simulink model "thermal_closed_loop_model"  (R2023a)
settings: Solver=ode23t  StartTime=0.0  StopTime=600  RelTol=1e-3
PostLoadFcn:
  | run('thermal_model_parameters.m')
  | run('thermal_harness_parameters.m')
  | run('thermal_variants_config.m')
values from neighbouring files (symbols this model uses):
  air_cp = 1004    [cathode_subsystem_parameters.m]    (also in thermal_subsystem_parameters.m)
  air_HC_min = 10    [cathode_subsystem_parameters.m]    (also in thermal_subsystem_parameters.m)
  air_HC_nom = 100    [cathode_subsystem_parameters.m]    (also in thermal_subsystem_parameters.m)
  air_rho = 1.2    [cathode_subsystem_parameters.m]    (also in thermal_subsystem_parameters.m)
  air_vel_nom = 1    [cathode_subsystem_parameters.m]    (also in thermal_subsystem_parameters.m)
  coolant_initial_pressure = 0.111325    [cathode_subsystem_parameters.m]    (also in thermal_subsystem_parameters.m)
  coolant_initial_temperature = 293.15    [cathode_subsystem_parameters.m]    (also in thermal_subsystem_parameters.m)
  coolant_tube_D = 0.05    [cathode_subsystem_parameters.m]    (also in thermal_subsystem_parameters.m)
  Hydrowell_VTS =     [Hydrowell_values_VLV.mat]
  radiator_area_air = 0.10260000000000001    (= 0.1026)    [cathode_subsystem_parameters.m]    (also in thermal_subsystem_parameters.m)
  radiator_area_fins = 2.5436250000000005    (= 2.543625)    [cathode_subsystem_parameters.m]    (also in thermal_subsystem_parameters.m)
  radiator_area_primary = 0.44452500000000011    (= 0.444525)    [cathode_subsystem_parameters.m]    (also in thermal_subsystem_parameters.m = 2 * radiator_tube_length * radiator_width * (radiator_fin_ro)
  radiator_n_tubes = 20    [cathode_subsystem_parameters.m]    (also in thermal_subsystem_parameters.m)
  radiator_tube_height = 0.0015    [cathode_subsystem_parameters.m]    (also in thermal_subsystem_parameters.m)
  radiator_tube_length = 0.45    [cathode_subsystem_parameters.m]    (also in thermal_subsystem_parameters.m)
  radiator_width = 0.025    [cathode_subsystem_parameters.m]    (also in thermal_subsystem_parameters.m)
  tcp_time_constant = 2    [cathode_subsystem_parameters.m]    (also in thermal_subsystem_parameters.m)
undefined symbols (not defined in the file or in its folder): sigbuilder_block, stack
libraries: fl_lib x153, nesl_utility x122, SimscapeFluids_lib x16, slpidlib x5, simulink x1
(part 8 of 8)

== system thermal_closed_loop_model/Plant Model H175-Cathode-S1/Sensor LH2 in ==
  Absolute Reference (2P) : fl_lib/Two-Phase Fluid/Elements/Absolute Reference (2P)
  Mass & Energy Flow Rate Sensor (2P)1 : fl_lib/Two-Phase Fluid/Sensors/Flow Rate Sensor (2P)  mass_flow_measure=true  volumetric_flow_measure=false  energy_flow_measure=true
      settings: InternalSimscapePortConfiguration="{\"Bottom\":[{\"id\":\"PHI\",\"label\":\"φ\",\"type\":\"output\"}],\"Left\":[{\"id\":\"A\",\"label\":\"A\",\"type\":\"foundation.two_phase_fluid.two_phase_fluid\"}],\"Right\":[{\"id\":\"B\",\"label\":\"B\",\"type\":\"foundation.two_phase_fluid.two_phase_fluid\"},{\"id\":\"M\",\"label\":\"M\",\"type\":\"output\"}],\"Top\":[]}"
  PS-Simulink Converter : nesl_utility/PS-Simulink Converter  PhysicalDomain=network_engine_domain  SubClassName=ps_output  LeftPortType=input  RightPortType=output  PseudoPeriodic=off  Frequencies=[]  VectorFormat=inherit  Unit=kW  AffineConversion=off
  PS-Simulink Converter1 : nesl_utility/PS-Simulink Converter  PhysicalDomain=network_engine_domain  SubClassName=ps_output  LeftPortType=input  RightPortType=output  PseudoPeriodic=off  Frequencies=[]  VectorFormat=1-D array  Unit=inherit  AffineConversion=off
  PS-Simulink Converter2 : nesl_utility/PS-Simulink Converter  PhysicalDomain=network_engine_domain  SubClassName=ps_output  LeftPortType=input  RightPortType=output  PseudoPeriodic=off  Frequencies=[]  VectorFormat=1-D array  Unit=inherit  AffineConversion=off
  PS-Simulink Converter3 : nesl_utility/PS-Simulink Converter  PhysicalDomain=network_engine_domain  SubClassName=ps_output  LeftPortType=input  RightPortType=output  PseudoPeriodic=off  Frequencies=[]  VectorFormat=1-D array  Unit=inherit  AffineConversion=off
  Pressure & Internal Energy Sensor (2P) : fl_lib/Two-Phase Fluid/Sensors/Pressure, Temperature & Internal Energy Sensor (2P)  reference=foundation.enum.MeasurementReference.difference  pressure=true  pressure_spec=foundation.enum.PressureMeasementSpec.Absolute  temperature=false  internal_energy=true
      settings: InternalSimscapePortConfiguration="{\"Bottom\":[{\"id\":\"U\",\"label\":\"U\",\"type\":\"output\"}],\"Left\":[{\"id\":\"A\",\"label\":\"A\",\"type\":\"foundation.two_phase_fluid.two_phase_fluid\"}],\"Right\":[{\"id\":\"B\",\"label\":\"B\",\"type\":\"foundation.two_phase_fluid.two_phase_fluid\"},{\"id\":\"P\",\"label\":\"P\",\"type\":\"output\"}],\"Top\":[]}"
  Thermodynamic Properties Sensor (2P) : fl_lib/Two-Phase Fluid/Sensors/Thermodynamic Properties Sensor (2P)  temperature=true  enthalpy=true  density=false  specific_volume=true  entropy=true
      settings: InternalSimscapePortConfiguration="{\"Bottom\":[{\"id\":\"V\",\"label\":\"v\",\"type\":\"output\"},{\"id\":\"S\",\"label\":\"s\",\"type\":\"output\"}],\"Left\":[{\"id\":\"A\",\"label\":\"A\",\"type\":\"foundation.two_phase_fluid.two_phase_fluid\"}],\"Right\":[{\"id\":\"T\",\"label\":\"T\",\"type\":\"output\"},{\"id\":\"H\",\"label\":\"h\",\"type\":\"output\"}],\"Top\":[]}"
  A : PMIOPort  Side=Left
  B : PMIOPort  Port=2  Side=Right
  tag scope: S5_Energy=global, S5_Temp=global, S5_aPres=global, S5_mFLow=global
  wires:
  PS-Simulink Converter3/1 -> [S5_mFLow]
  PS-Simulink Converter2/1 -> [S5_aPres]
  PS-Simulink Converter1/1 -> [S5_Temp]
  PS-Simulink Converter/1 -> [S5_Energy]
  connections:
  Pressure & Internal Energy Sensor (2P)/RConn1 -- Absolute Reference (2P)/LConn1
  Mass & Energy Flow Rate Sensor (2P)1/RConn2 -- PS-Simulink Converter3/LConn1
  PS-Simulink Converter2/LConn1 -- Pressure & Internal Energy Sensor (2P)/RConn2
  Thermodynamic Properties Sensor (2P)/RConn1 -- PS-Simulink Converter1/LConn1
  Mass & Energy Flow Rate Sensor (2P)1/RConn3 -- PS-Simulink Converter/LConn1
  Mass & Energy Flow Rate Sensor (2P)1/LConn1 -- Pressure & Internal Energy Sensor (2P)/LConn1 -- Thermodynamic Properties Sensor (2P)/LConn1 -- A/RConn1
  Mass & Energy Flow Rate Sensor (2P)1/RConn1 -- B/RConn1

== system thermal_closed_loop_model/Plant Model H175-Cathode-S1/Sensor LH2 out ==
  Absolute Reference (2P) : fl_lib/Two-Phase Fluid/Elements/Absolute Reference (2P)
  Mass & Energy Flow Rate Sensor (2P)1 : fl_lib/Two-Phase Fluid/Sensors/Flow Rate Sensor (2P)  mass_flow_measure=true  volumetric_flow_measure=false  energy_flow_measure=true
      settings: InternalSimscapePortConfiguration="{\"Bottom\":[{\"id\":\"PHI\",\"label\":\"φ\",\"type\":\"output\"}],\"Left\":[{\"id\":\"A\",\"label\":\"A\",\"type\":\"foundation.two_phase_fluid.two_phase_fluid\"}],\"Right\":[{\"id\":\"B\",\"label\":\"B\",\"type\":\"foundation.two_phase_fluid.two_phase_fluid\"},{\"id\":\"M\",\"label\":\"M\",\"type\":\"output\"}],\"Top\":[]}"
  PS-Simulink Converter : nesl_utility/PS-Simulink Converter  PhysicalDomain=network_engine_domain  SubClassName=ps_output  LeftPortType=input  RightPortType=output  PseudoPeriodic=off  Frequencies=[]  VectorFormat=1-D array  Unit=kW  AffineConversion=off
  PS-Simulink Converter1 : nesl_utility/PS-Simulink Converter  PhysicalDomain=network_engine_domain  SubClassName=ps_output  LeftPortType=input  RightPortType=output  PseudoPeriodic=off  Frequencies=[]  VectorFormat=1-D array  Unit=degC  AffineConversion=off
  PS-Simulink Converter2 : nesl_utility/PS-Simulink Converter  PhysicalDomain=network_engine_domain  SubClassName=ps_output  LeftPortType=input  RightPortType=output  PseudoPeriodic=off  Frequencies=[]  VectorFormat=1-D array  Unit=1  AffineConversion=off
  PS-Simulink Converter3 : nesl_utility/PS-Simulink Converter  PhysicalDomain=network_engine_domain  SubClassName=ps_output  LeftPortType=input  RightPortType=output  PseudoPeriodic=off  Frequencies=[]  VectorFormat=1-D array  Unit=inherit  AffineConversion=off
  Pressure & Internal Energy Sensor (2P) : fl_lib/Two-Phase Fluid/Sensors/Pressure, Temperature & Internal Energy Sensor (2P)  reference=foundation.enum.MeasurementReference.difference  pressure=true  pressure_spec=foundation.enum.PressureMeasementSpec.Absolute  temperature=false  internal_energy=true
      settings: InternalSimscapePortConfiguration="{\"Bottom\":[{\"id\":\"U\",\"label\":\"U\",\"type\":\"output\"}],\"Left\":[{\"id\":\"A\",\"label\":\"A\",\"type\":\"foundation.two_phase_fluid.two_phase_fluid\"}],\"Right\":[{\"id\":\"B\",\"label\":\"B\",\"type\":\"foundation.two_phase_fluid.two_phase_fluid\"},{\"id\":\"P\",\"label\":\"P\",\"type\":\"output\"}],\"Top\":[]}"
  Thermodynamic Properties Sensor (2P) : fl_lib/Two-Phase Fluid/Sensors/Thermodynamic Properties Sensor (2P)  temperature=true  enthalpy=true  density=false  specific_volume=true  entropy=true
      settings: InternalSimscapePortConfiguration="{\"Bottom\":[{\"id\":\"V\",\"label\":\"v\",\"type\":\"output\"},{\"id\":\"S\",\"label\":\"s\",\"type\":\"output\"}],\"Left\":[{\"id\":\"A\",\"label\":\"A\",\"type\":\"foundation.two_phase_fluid.two_phase_fluid\"}],\"Right\":[{\"id\":\"T\",\"label\":\"T\",\"type\":\"output\"},{\"id\":\"H\",\"label\":\"h\",\"type\":\"output\"}],\"Top\":[]}"
  A : PMIOPort  Side=Left
  B : PMIOPort  Port=2  Side=Right
  tag scope: S6_Energy=global, S6_Temp=global, S6_aPres=global, S6_mFlow=global
  wires:
  PS-Simulink Converter3/1 -> [S6_aPres]
  PS-Simulink Converter2/1 -> [S6_mFlow]
  PS-Simulink Converter/1 -> [S6_Energy]
  PS-Simulink Converter1/1 -> [S6_Temp]
  connections:
  Pressure & Internal Energy Sensor (2P)/RConn1 -- Absolute Reference (2P)/LConn1
  Mass & Energy Flow Rate Sensor (2P)1/LConn1 -- Pressure & Internal Energy Sensor (2P)/LConn1 -- Thermodynamic Properties Sensor (2P)/LConn1 -- A/RConn1
  Pressure & Internal Energy Sensor (2P)/RConn2 -- PS-Simulink Converter3/LConn1
  Mass & Energy Flow Rate Sensor (2P)1/RConn2 -- PS-Simulink Converter2/LConn1
  Thermodynamic Properties Sensor (2P)/RConn1 -- PS-Simulink Converter1/LConn1
  Mass & Energy Flow Rate Sensor (2P)1/RConn1 -- B/RConn1
  Mass & Energy Flow Rate Sensor (2P)1/RConn3 -- PS-Simulink Converter/LConn1

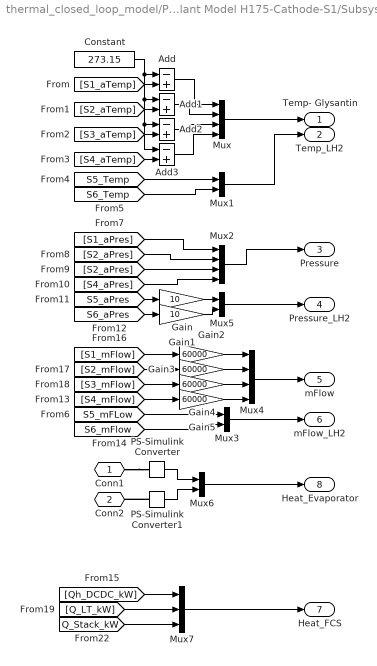
== system thermal_closed_loop_model/Plant Model H175-Cathode-S1/Subsystem4 ==
  Add{,1..3} (4 alike) : Sum  Inputs=-+
  Constant : Constant  Value=273.15
  Gain : Gain  Gain=10
  Gain1 : Gain  Gain=10
  Gain{2..5} (4 alike) : Gain  Gain=60000
  Mux : Mux
  Mux{1,3,5..6} (4 alike) : Mux  Inputs=2
  Mux2 : Mux
  Mux4 : Mux
  Mux7 : Mux  Inputs=3
  PS-Simulink Converter : nesl_utility/PS-Simulink Converter  PhysicalDomain=network_engine_domain  SubClassName=ps_output  LeftPortType=input  RightPortType=output  PseudoPeriodic=off  Frequencies=[]  VectorFormat=inherit  Unit=inherit  AffineConversion=off
  PS-Simulink Converter1 : nesl_utility/PS-Simulink Converter  PhysicalDomain=network_engine_domain  SubClassName=ps_output  LeftPortType=input  RightPortType=output  PseudoPeriodic=off  Frequencies=[]  VectorFormat=inherit  Unit=inherit  AffineConversion=off
  Conn1 : PMIOPort  Side=Left
  Conn2 : PMIOPort  Port=2  Side=Left
  Temp- Glysantin : Outport
  Temp_LH2 : Outport  Port=2
  Pressure : Outport  Port=3
  Pressure_LH2 : Outport  Port=4
  mFlow : Outport  Port=5
  mFlow_LH2 : Outport  Port=6
  Heat_FCS : Outport  Port=7
  Heat_Evaporator : Outport  Port=8
  wires:
  Mux7/1 -> Heat_FCS/1
  [Q_Stack_kW] -> Mux7/3
  [Q_LT_kW] -> Mux7/2
  [Qh_DCDC_kW] -> Mux7/1
  Mux6/1 -> Heat_Evaporator/1
  PS-Simulink Converter1/1 -> Mux6/2
  PS-Simulink Converter/1 -> Mux6/1
  Gain5/1 -> Mux4/4
  Gain4/1 -> Mux4/3
  Gain3/1 -> Mux4/2
  Gain2/1 -> Mux4/1
  Gain1/1 -> Mux5/2
  Gain/1 -> Mux5/1
  [S5_aPres] -> Gain/1
  Mux5/1 -> Pressure_LH2/1
  [S6_aPres] -> Gain1/1
  Mux3/1 -> mFlow_LH2/1
  [S5_mFLow] -> Mux3/1
  Add/1 -> Mux/1
  Add1/1 -> Mux/2
  Add2/1 -> Mux/3
  Add3/1 -> Mux/4
  [S5_Temp] -> Mux1/1
  [S6_Temp] -> Mux1/2
  [S4_aTemp] -> Add3/2
  [S3_aTemp] -> Add2/2
  [S2_aTemp] -> Add1/2
  Constant/1 -> Add/1, Add1/1, Add2/1, Add3/1
  [S1_aTemp] -> Add/2
  Mux2/1 -> Pressure/1
  Mux1/1 -> Temp_LH2/1
  Mux/1 -> Temp- Glysantin/1
  Mux4/1 -> mFlow/1
  [S6_mFlow] -> Mux3/2
  [S1_aPres] -> Mux2/1
  [S4_mFlow] -> Gain5/1
  [S2_aPres] -> Mux2/2
  [S3_mFlow] -> Gain4/1
  [S2_aPres] -> Mux2/3
  [S1_mFlow] -> Gain2/1
  [S2_mFlow] -> Gain3/1
  [S4_aPres] -> Mux2/4
  connections:
  PS-Simulink Converter1/LConn1 -- Conn2/RConn1
  Conn1/RConn1 -- PS-Simulink Converter/LConn1

== system thermal_closed_loop_model/Plant_Sensors1/EAC_Theo_Power ==
  <mFlow_S1> : Inport
  <aPres_S1> : Inport  Port=2
  <aPres_S2> : Inport  Port=3
  <aTemp_S1> : Inport  Port=4
  Cp : Constant  Value=1004
  Divide : Product  Inputs=*/
  MATLAB Function : MATLAB Function  TreatAsAtomicUnit=on
  Product : Product  Inputs=4
  y-exp : Constant  Value=(1.33-1)/1.33
  Out1 : Outport
  wires:
  Cp/1 -> Product/1
  <aTemp_S1>/1 -> Product/2
  <aPres_S1>/1 -> Divide/2
  Product/1 -> Out1/1
  <aPres_S2>/1 -> Divide/1
  MATLAB Function/1(y) -> Product/4
  y-exp/1 -> MATLAB Function/2(data)
  Divide/1 -> MATLAB Function/1(u)
  <mFlow_S1>/1 -> Product/3

== system thermal_closed_loop_model/Plant_Sensors1/EAT_Theo_Power ==
  <mFlow_S1> : Inport
  <aPres_S6> : Inport  Port=2
  <aTemp_S6> : Inport  Port=3
  <aPres_S7> : Inport  Port=4
  Cp : Constant  Value=1150
  Divide : Product  Inputs=*/
  Gain : Gain  Gain=-1
  MATLAB Function : MATLAB Function  TreatAsAtomicUnit=on
  Product : Product  Inputs=4
  y-exp : Constant  Value=(1.33-1)/1.33
  Out1 : Outport
  wires:
  y-exp/1 -> MATLAB Function/2(data)
  <aPres_S7>/1 -> Divide/1
  Cp/1 -> Product/4
  Divide/1 -> MATLAB Function/1(u)
  Product/1 -> Gain/1
  <mFlow_S1>/1 -> Product/2
  MATLAB Function/1(y) -> Product/1
  <aTemp_S6>/1 -> Product/3
  <aPres_S6>/1 -> Divide/2
  Gain/1 -> Out1/1

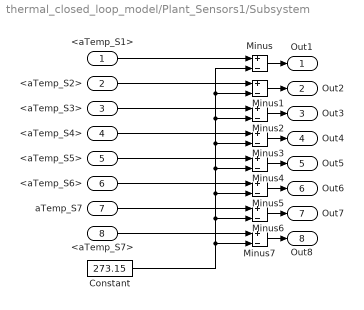
== system thermal_closed_loop_model/Plant_Sensors1/Subsystem ==
  <aTemp_S1> : Inport
  <aTemp_S2> : Inport  Port=2
  <aTemp_S3> : Inport  Port=3
  <aTemp_S4> : Inport  Port=4
  <aTemp_S5> : Inport  Port=5
  <aTemp_S6> : Inport  Port=6
  aTemp_S7 : Inport  Port=7
  <aTemp_S7> : Inport  Port=8
  Constant : Constant  Value=273.15
  Minus{,1..7} (8 alike) : Sum  Inputs=+-
  Out1 : Outport
  Out2 : Outport  Port=2
  Out3 : Outport  Port=3
  Out4 : Outport  Port=4
  Out5 : Outport  Port=5
  Out6 : Outport  Port=6
  Out7 : Outport  Port=7
  Out8 : Outport  Port=8
  wires:
  Minus4/1 -> Out5/1
  Constant/1 -> Minus7/2, Minus3/2, Minus2/2, Minus1/2, Minus/2, Minus4/2, Minus5/2, Minus6/2
  Minus2/1 -> Out3/1
  <aTemp_S7>/1 -> Minus7/1
  <aTemp_S4>/1 -> Minus3/1
  <aTemp_S1>/1 -> Minus/1
  Minus5/1 -> Out6/1
  Minus6/1 -> Out7/1
  <aTemp_S3>/1 -> Minus2/1
  Minus/1 -> Out1/1
  <aTemp_S5>/1 -> Minus4/1
  Minus3/1 -> Out4/1
  Minus1/1 -> Out2/1
  <aTemp_S6>/1 -> Minus5/1
  <aTemp_S2>/1 -> Minus1/1
  Minus7/1 -> Out8/1
  aTemp_S7/1 -> Minus6/1

== system thermal_closed_loop_model/Basic Peripherals/Variant Subsystem/Controlled_Power_HeatExchanger ==
  note: Lafer-style heat exchanger
  Environment_Temperature_K : Inport
  Heat_Flux_W : Inport  Port=2
  Controlled Temperature Source : fl_lib/Thermal/Thermal Sources/Controlled Temperature Source
  Controlled Heat Flow Rate Source : fl_lib/Thermal/Thermal Sources/Controlled Heat Flow Rate Source
  Gain : Gain  Gain=-1
  Heat Exchanger Interface (TL) : SimscapeFluids_lib/Fluid Network Interfaces/Heat Exchangers/Fundamental Components/Heat Exchanger Interface (TL)  min_flow_area=radiator_n_tubes*(radiator_width*radiator_tube_height) m^2  Dh_press=4*(radiator_width*radiator_tube_height)/(2 * (radiator_width+radiator_tube_height)) m  liquid_volume=radiator_n_tubes*(radiator_width*radiator_tube_height)*radiator_tube_length m^3  Re_lam=2000  Re_tur=4000.  pressure_loss_spec=fluids.interfaces.enum.pressure_loss_spec.tube_correlation  pressure_loss_coeff=0.1  length_press=radiator_tube_length m  length_add=0.1 m  roughness=15e-6 m  Re_friction_TLU=[400, 1000, 1500, 3000, 4000, 6000, 10000, 20000, 40000, 60000, 100000, 100000000]  friction_factor_TLU=[.264, .112, .071, .0417, .0387, .0268, .025, .0232, .0226, .022, .0214, .0214]  shape_factor=64  Re_Euler_TLU=[50, 500, 1000, 2000]  Euler_TLU=[4.4505, .6864, .4791, .3755]  heat_transfer_spec=fluids.interfaces.enum.heat_transfer_spec.tube_correlation  heat_coeff=100 W/(K*m^2)  heat_transfer_area=radiator_n_tubes*2*(radiator_tube_length*radiator_width+radiator_tube_length*radiator_tube_height) m^2  Nu_lam=3.66  Re_Colburn_TLU=[100, 150, 1000]  Colburn_factor_TLU=[.019, .013, .002]  Re_Nu_TLU=[100, 150, 1000]  Pr_Nu_TLU=[1, 10]  Nu_TLU=[3.72, 4.21; 3.75, 4.44; 4.21, 7.15]  length_heat=radiator_tube_length m  dynamic_compressibility=simscape.enum.onoff.on  T0=coolant_initial_temperature K  p0=coolant_initial_pressure MPa
      settings: InternalSimscapePortConfiguration="{\"Bottom\":[],\"Left\":[{\"id\":\"A\",\"label\":\"A\",\"type\":\"foundation.thermal_liquid.thermal_liquid\"},{\"id\":\"B\",\"label\":\"B\",\"type\":\"foundation.thermal_liquid.thermal_liquid\"}],\"Right\":[{\"id\":\"H\",\"label\":\"H\",\"type\":\"foundation.thermal.thermal\"},{\"id\":\"C\",\"label\":\"C\",\"type\":\"output\"},{\"id\":\"HC\",\"label\":\"HC\",\"type\":\"output\"}],\"Top\":[]}"
  PS Terminator : fl_lib/Physical Signals/Sinks/PS Terminator
  PS Terminator1 : fl_lib/Physical Signals/Sinks/PS Terminator
  Saturation : Saturate  UpperLimit=0  LowerLimit=-200e3
  Simulink-PS Converter3 : nesl_utility/Simulink-PS Converter  PhysicalDomain=network_engine_domain  SubClassName=ps_input  LeftPortType=input  RightPortType=output  PseudoPeriodic=off  Frequencies=[]  NoiseDistribution=none  NoiseParameters=[]  Unit=1  AffineConversion=off  FilteringAndDerivatives=provide  SimscapeFilterOrder=1  InputFilterTimeConstant=0.001  UdotUserProvided=0
  Simulink-PS Converter5 : nesl_utility/Simulink-PS Converter  PhysicalDomain=network_engine_domain  SubClassName=ps_input  LeftPortType=input  RightPortType=output  PseudoPeriodic=off  Frequencies=[]  NoiseDistribution=none  NoiseParameters=[]  Unit=1  AffineConversion=off  FilteringAndDerivatives=provide  SimscapeFilterOrder=1  InputFilterTimeConstant=0.001  UdotUserProvided=0
  Thermal Reference : fl_lib/Thermal/Thermal Elements/Thermal Reference
  Coolant_to_HeatExchanger : PMIOPort  Side=Right
  Coolant_from_HeatExchanger : PMIOPort  Port=2  Side=Right
  wires:
  Environment_Temperature_K/1 -> Simulink-PS Converter5/1
  Heat_Flux_W/1 -> Gain/1
  Gain/1 -> Saturation/1
  Saturation/1 -> Simulink-PS Converter3/1
  connections:
  Coolant_to_HeatExchanger/RConn1 -- Heat Exchanger Interface (TL)/LConn1
  PS Terminator/LConn1 -- Heat Exchanger Interface (TL)/RConn2
  Controlled Heat Flow Rate Source/RConn2 -- Controlled Temperature Source/LConn1
  Controlled Temperature Source/RConn2 -- Thermal Reference/LConn1
  Controlled Heat Flow Rate Source/LConn1 -- Heat Exchanger Interface (TL)/RConn1
  Simulink-PS Converter3/RConn1 -- Controlled Heat Flow Rate Source/RConn1
  PS Terminator1/LConn1 -- Heat Exchanger Interface (TL)/RConn3
  Simulink-PS Converter5/RConn1 -- Controlled Temperature Source/RConn1
  Coolant_from_HeatExchanger/RConn1 -- Heat Exchanger Interface (TL)/LConn2

== system thermal_closed_loop_model/Basic Peripherals/Variant Subsystem/Controlled_Temperature_HeatExchanger ==
  note: Lafer-style heat exchanger
  T_TCVi_ref_degC : Inport
  Controlled Temperature Source : fl_lib/Thermal/Thermal Sources/Controlled Temperature Source
  Controlled Heat Flow Rate Source : fl_lib/Thermal/Thermal Sources/Controlled Heat Flow Rate Source
  Gain : Gain  Gain=-20e3
  Heat Exchanger Interface (TL) : SimscapeFluids_lib/Fluid Network Interfaces/Heat Exchangers/Fundamental Components/Heat Exchanger Interface (TL)  min_flow_area=radiator_n_tubes*(radiator_width*radiator_tube_height) m^2  Dh_press=4*(radiator_width*radiator_tube_height)/(2 * (radiator_width+radiator_tube_height)) m  liquid_volume=radiator_n_tubes*(radiator_width*radiator_tube_height)*radiator_tube_length m^3  Re_lam=2000  Re_tur=4000.  pressure_loss_spec=fluids.interfaces.enum.pressure_loss_spec.tube_correlation  pressure_loss_coeff=0.1  length_press=radiator_tube_length m  length_add=0.1 m  roughness=15e-6 m  Re_friction_TLU=[400, 1000, 1500, 3000, 4000, 6000, 10000, 20000, 40000, 60000, 100000, 100000000]  friction_factor_TLU=[.264, .112, .071, .0417, .0387, .0268, .025, .0232, .0226, .022, .0214, .0214]  shape_factor=64  Re_Euler_TLU=[50, 500, 1000, 2000]  Euler_TLU=[4.4505, .6864, .4791, .3755]  heat_transfer_spec=fluids.interfaces.enum.heat_transfer_spec.tube_correlation  heat_coeff=100 W/(K*m^2)  heat_transfer_area=radiator_n_tubes*2*(radiator_tube_length*radiator_width+radiator_tube_length*radiator_tube_height) m^2  Nu_lam=3.66  Re_Colburn_TLU=[100, 150, 1000]  Colburn_factor_TLU=[.019, .013, .002]  Re_Nu_TLU=[100, 150, 1000]  Pr_Nu_TLU=[1, 10]  Nu_TLU=[3.72, 4.21; 3.75, 4.44; 4.21, 7.15]  length_heat=radiator_tube_length m  dynamic_compressibility=simscape.enum.onoff.on  T0=coolant_initial_temperature K  p0=coolant_initial_pressure MPa
      settings: InternalSimscapePortConfiguration="{\"Bottom\":[],\"Left\":[{\"id\":\"A\",\"label\":\"A\",\"type\":\"foundation.thermal_liquid.thermal_liquid\"},{\"id\":\"B\",\"label\":\"B\",\"type\":\"foundation.thermal_liquid.thermal_liquid\"}],\"Right\":[{\"id\":\"H\",\"label\":\"H\",\"type\":\"foundation.thermal.thermal\"},{\"id\":\"C\",\"label\":\"C\",\"type\":\"output\"},{\"id\":\"HC\",\"label\":\"HC\",\"type\":\"output\"}],\"Top\":[]}"
  PS Terminator : fl_lib/Physical Signals/Sinks/PS Terminator
  PS Terminator1 : fl_lib/Physical Signals/Sinks/PS Terminator
  PS-Simulink Converter : nesl_utility/PS-Simulink Converter  PhysicalDomain=network_engine_domain  SubClassName=ps_output  LeftPortType=input  RightPortType=output  PseudoPeriodic=off  Frequencies=[]  VectorFormat=inherit  Unit=inherit  AffineConversion=off
  Pressure & Temperature Sensor (TL)1 : fl_lib/Thermal Liquid/Sensors/Pressure & Temperature Sensor (TL)  reference=foundation.enum.MeasurementReference.absolute  pressure=false  pressure_spec=foundation.enum.PressureMeasementSpec.Absolute  temperature=true
      settings: InternalSimscapePortConfiguration="{\"Bottom\":[{\"id\":\"T\",\"label\":\"T\",\"type\":\"output\"}],\"Left\":[{\"id\":\"A\",\"label\":\"A\",\"type\":\"foundation.thermal_liquid.thermal_liquid\"}],\"Right\":[],\"Top\":[]}"
  Saturation : Saturate  UpperLimit=0  LowerLimit=-200e3
  Simulink-PS Converter3 : nesl_utility/Simulink-PS Converter  PhysicalDomain=network_engine_domain  SubClassName=ps_input  LeftPortType=input  RightPortType=output  PseudoPeriodic=off  Frequencies=[]  NoiseDistribution=none  NoiseParameters=[]  Unit=1  AffineConversion=off  FilteringAndDerivatives=provide  SimscapeFilterOrder=1  InputFilterTimeConstant=0.001  UdotUserProvided=0
  Simulink-PS Converter5 : nesl_utility/Simulink-PS Converter  PhysicalDomain=network_engine_domain  SubClassName=ps_input  LeftPortType=input  RightPortType=output  PseudoPeriodic=off  Frequencies=[]  NoiseDistribution=none  NoiseParameters=[]  Unit=1  AffineConversion=off  FilteringAndDerivatives=provide  SimscapeFilterOrder=1  InputFilterTimeConstant=0.001  UdotUserProvided=0
  Sum : Sum  Inputs=|+-
  Thermal Reference : fl_lib/Thermal/Thermal Elements/Thermal Reference
  Unit Delay17 : UnitDelay  SampleTime=-1  HasFrameUpgradeWarning=on
  °C to Kelvin : Subsystem
  Coolant_to_HeatExchanger : PMIOPort  Side=Right
  Coolant_from_HeatExchanger : PMIOPort  Port=2  Side=Right
  tag scope: T_TCVi_ref_degC=global
  wires:
  PS-Simulink Converter/1 -> Sum/1
  Gain/1 -> Unit Delay17/1
  Unit Delay17/1 -> Saturation/1
  T_TCVi_ref_degC/1 -> [T_TCVi_ref_degC], °C to Kelvin/1(Temp. (°C))
  Sum/1 -> Gain/1
  Saturation/1 -> Simulink-PS Converter3/1
  °C to Kelvin/1(Temp. (K)) -> Simulink-PS Converter5/1, Sum/2  "Stack Inlet Temperature: TSens_CLSti 6812 (°C)"
  connections:
  Coolant_from_HeatExchanger/RConn1 -- Pressure & Temperature Sensor (TL)1/LConn1 -- Heat Exchanger Interface (TL)/LConn2
  Simulink-PS Converter5/RConn1 -- Controlled Temperature Source/RConn1
  PS Terminator1/LConn1 -- Heat Exchanger Interface (TL)/RConn3
  Simulink-PS Converter3/RConn1 -- Controlled Heat Flow Rate Source/RConn1
  Controlled Heat Flow Rate Source/LConn1 -- Heat Exchanger Interface (TL)/RConn1
  Controlled Temperature Source/RConn2 -- Thermal Reference/LConn1
  PS-Simulink Converter/LConn1 -- Pressure & Temperature Sensor (TL)1/RConn1
  Controlled Heat Flow Rate Source/RConn2 -- Controlled Temperature Source/LConn1
  PS Terminator/LConn1 -- Heat Exchanger Interface (TL)/RConn2
  Heat Exchanger Interface (TL)/LConn1 -- Coolant_to_HeatExchanger/RConn1

== system thermal_closed_loop_model/Basic Peripherals/Variant Subsystem/Phyiscal_Radiator_Model ==
  note: Basic Radiator Model
  Convective_Airspeed_mps : Inport
  Environment_Temperature_K : Inport  Port=2
  Aircraft Duct : Subsystem
  Radiator : SimscapeFluids_lib/Fluid Network Interfaces/Heat Exchangers/Heat Exchanger (TL)  hex_type=3  shell_num=1  cross_type=4  NTU_TLU=[0.5, 1.0, 2.0, 3.0, 4.0, 5.0]  CR_TLU=[0.0, 0.25, 0.5, 0.75, 1.0]  eff_TLU=[0.3, 0.3, 0.3, 0.3, 0.3; 0.6, 0.55, 0.5, 0.47, 0.43; 0.85, 0.76, 0.68, 0.61, 0.55; 0.94, 0.83, 0.72, 0.65, 0.58; 0.98, 0.86, 0.75, 0.66, 0.58; 0.99, 0.86, 0.75, 0.66, 0.58]  R_wall=0.014/(381*radiator_n_tubes*radiator_width*radiator_tube_length) K/W  min_flow_area_1=radiator_n_tubes*(radiator_width*radiator_tube_height) m^2  Dh_press_1=4*(radiator_width*radiator_tube_height)/(2 * (radiator_width+radiator_tube_height)) m  liquid_volume_1=radiator_n_tubes*(radiator_width*radiator_tube_height)*radiator_tube_length m^3  Re_lam_1=2000  Re_tur_1=4000  pressure_loss_spec_1=fluids.interfaces.enum.pressure_loss_spec.tube_correlation  pressure_loss_coeff_1=15  length_press_1=radiator_tube_length m  length_add_1=0.1 m  roughness_1=15e-6 m  Re_friction_TLU_1=[400.0, 1000.0, 1500.0, 3000.0, 4000.0, 6000.0, 10000.0, 20000.0, 40000.0, 60000.0, 100000.0, 100000000.0]  friction_factor_TLU_1=[0.264, 0.112, 0.071, 0.0417, 0.0387, 0.0268, 0.025, 0.0232, 0.0226, 0.022, 0.0214, 0.0214]  shape_factor_1=64  Re_Euler_TLU_1=[50.0, 500.0, 1000.0, 2000.0]  Euler_TLU_1=[4.4505, 0.6864, 0.4791, 0.3755]  heat_transfer_spec_1=2  heat_transfer_area_1=radiator_n_tubes*2*(radiator_tube_length*radiator_width+radiator_tube_length*radiator_tube_height) m^2  heat_coeff_1=2000 W/(m^2 * K)  length_heat_1=radiator_tube_length cm  Nu_lam_1=3.66  Re_Colburn_TLU_1=[100.0, 150.0, 1000.0]  Colburn_factor_TLU_1=[0.019, 0.013, 0.002]  Re_Nu_TLU_1=[100.0, 150.0, 1000.0]  Pr_Nu_TLU_1=[1.0, 10.0]  Nu_TLU_1=[3.72, 4.21; 3.75, 4.44; 4.21, 7.15]  fouling_factor_1=0 m^2*K/W  min_heat_coeff_1=5 W/(m^2 * K)  heat_transfer_area_2=radiator_area_primary+radiator_area_fins m^2  fouling_factor_2=0 m^2*K/W  min_heat_coeff_2=0.01 W/(m^2 * K)  dynamic_compressibility_1=1  T0_1=coolant_initial_temperature K  p0_1=coolant_initial_pressure MPa  mdot1_TLU=[.1, .2] kg/s  mdot2_TLU=[.2, .3] kg/s  SD_TLU=[35, 35; 50, 50] kW/K  Q_check=1  mdot_dp_TLU_1=[.1, .2] kg/s  p_diff_TLU_1=[.003, .005] MPa  T_ref_in_1=293.15 K  p_ref_in_1=0.101325 MPa  mdot_threshold_1=1e-3 kg/s  area_1=0.01 m^2
      settings: InternalSimscapePortConfiguration="{\"Bottom\":[],\"Left\":[{\"id\":\"A1\",\"label\":\"A1\",\"type\":\"foundation.thermal_liquid.thermal_liquid\"},{\"id\":\"B1\",\"label\":\"B1\",\"type\":\"foundation.thermal_liquid.thermal_liquid\"}],\"Right\":[{\"id\":\"H2\",\"label\":\"H2\",\"type\":\"foundation.thermal.thermal\"},{\"id\":\"C2\",\"label\":\"C2\",\"type\":\"input\"},{\"id\":\"HC2\",\"label\":\"HC2\",\"type\":\"input\"}],\"Top\":[]}"
  Coolant_to_HeatExchanger : PMIOPort  Side=Right
  Coolant_from_HeatExchanger : PMIOPort  Port=2  Side=Right
  wires:
  Environment_Temperature_K/1 -> Aircraft Duct/2(T_air)
  Convective_Airspeed_mps/1 -> Aircraft Duct/1(V_air)
  connections:
  Radiator/RConn1 -- Aircraft Duct/RConn1
  Radiator/RConn2 -- Aircraft Duct/RConn2
  Radiator/LConn1 -- Coolant_to_HeatExchanger/RConn1
  Radiator/RConn3 -- Aircraft Duct/RConn3
  Coolant_from_HeatExchanger/RConn1 -- Radiator/LConn2

== system thermal_closed_loop_model/Fast Controller/CHU-Dry side control/Cathode Humidifier ==
  Controlled Moisture Source (MA) : fl_lib/Moist Air/Sources/Moisture & Trace Gas Sources/Controlled Moisture Source (MA)  moisture_source_spec=foundation.enum.moisture_source_spec.vapor  Phi_S_specify=off  Phi_S_priority=None  Phi_S=0 kW  Phi_S_nominal_specify=off  Phi_S_nominal_unit=kW  Phi_S_nominal_value=1  mdot_w_S_specify=off  mdot_w_S_priority=None  mdot_w_S=0 kg/s  mdot_w_S_nominal_specify=off  mdot_w_S_nominal_unit=kg/s  mdot_w_S_nominal_value=1
      settings: InternalSimscapePortConfiguration="{\"Bottom\":[],\"Left\":[{\"id\":\"S\",\"label\":\"S\",\"type\":\"foundation.moist_air.moist_air_source\"}],\"Right\":[{\"id\":\"M\",\"label\":\"M\",\"type\":\"input\"},{\"id\":\"T\",\"label\":\"T\",\"type\":\"input\"}],\"Top\":[]}"
  Measurement Selector (MA) : fl_lib/Moist Air/Sensors/Measurement Selector (MA)  moisture_spec=foundation.enum.moisture_spec.relative_humidity  trace_gas_spec=foundation.enum.trace_gas_spec.mole_fraction
  PS-Simulink Converter : nesl_utility/PS-Simulink Converter  PhysicalDomain=network_engine_domain  SubClassName=ps_output  LeftPortType=input  RightPortType=output  PseudoPeriodic=off  Frequencies=[]  VectorFormat=1-D array  Unit=1  AffineConversion=off
  Perfect Insulator : fl_lib/Thermal/Thermal Elements/Perfect Insulator  T_specify=off  T_priority=None  T=0 K  T_nominal_specify=off  T_nominal_unit=K  T_nominal_value=1
  Pipe (MA) : fl_lib/Moist Air/Elements/Pipe (MA)  length=0.25 m  area=pi*0.05^2/4 m^2  Dh=0.05 m  length_add=0.1 m  roughness=15e-6 m  Re_lam=2000  Re_tur=4000  shape_factor=64  Nu_lam=3.66  wall_condensation=simscape.enum.onoff.off  RH_ws=1  time_constant=1e-3 s  moisture_trace_gas_source=foundation.enum.moisture_trace_gas_source.controlled  moisture_source_spec=foundation.enum.moisture_source_spec.vapor  moisture_mass_flow=0 kg/s  moisture_temperature_spec=foundation.enum.temperature_spec.atmospheric  moisture_temperature=293.15 K  trace_gas_mass_flow=0 kg/s  trace_gas_temperature_spec=foundation.enum.temperature_spec.atmospheric  trace_gas_temperature=293.15 K  p_I_specify=off  p_I_priority=High  p_I=env_p MPa  p_I_nominal_specify=off  p_I_nominal_unit=MPa  p_I_nominal_value=1  T_I_specify=off  T_I_priority=High  T_I=env_T degC  T_I_nominal_specify=off  T_I_nominal_unit=K  T_I_nominal_value=1  RH_I_specify=off  RH_I_priority=High  RH_I=env_RH  RH_I_nominal_specify=off  RH_I_nominal_unit=1  RH_I_nominal_value=1  x_w_I_specify=off  x_w_I_priority=None  x_w_I=0  x_w_I_nominal_specify=off  x_w_I_nominal_unit=1  x_w_I_nominal_value=1  y_w_I_specify=off  y_w_I_priority=None  y_w_I=0  y_w_I_nominal_specify=off  y_w_I_nominal_unit=1  y_w_I_nominal_value=1  HR_I_specify=off  HR_I_priority=None  HR_I=0  HR_I_nominal_specify=off  HR_I_nominal_unit=1  HR_I_nominal_value=1  x_g_I_specify=off  x_g_I_priority=None  x_g_I=0  x_g_I_nominal_specify=off  x_g_I_nominal_unit=1  x_g_I_nominal_value=1  y_g_I_specify=off  y_g_I_priority=High  y_g_I=env_yO2  y_g_I_nominal_specify=off  y_g_I_nominal_unit=1  y_g_I_nominal_value=1
      settings: InternalSimscapePortConfiguration="{\"Bottom\":[],\"Left\":[{\"id\":\"A\",\"label\":\"A\",\"type\":\"foundation.moist_air.moist_air\"},{\"id\":\"H\",\"label\":\"H\",\"type\":\"foundation.thermal.thermal\"},{\"id\":\"S\",\"label\":\"S\",\"type\":\"foundation.moist_air.moist_air_source\"}],\"Right\":[{\"id\":\"B\",\"label\":\"B\",\"type\":\"foundation.moist_air.moist_air\"},{\"id\":\"W\",\"label\":\"W\",\"type\":\"output\"},{\"id\":\"F\",\"label\":\"F\",\"type\":\"output\"}],\"Top\":[]}"
  Proportional Control : Subsystem
  Relative Humidity : Constant  Value=.76
  Simulink-PS Converter : nesl_utility/Simulink-PS Converter  PhysicalDomain=network_engine_domain  SubClassName=ps_input  LeftPortType=input  RightPortType=output  PseudoPeriodic=off  Frequencies=[]  NoiseDistribution=none  NoiseParameters=[]  Unit=kg/s  AffineConversion=off  FilteringAndDerivatives=provide  SimscapeFilterOrder=1  InputFilterTimeConstant=0.001  UdotUserProvided=0
  Simulink-PS Converter1 : nesl_utility/Simulink-PS Converter  PhysicalDomain=network_engine_domain  SubClassName=ps_input  LeftPortType=input  RightPortType=output  PseudoPeriodic=off  Frequencies=[]  NoiseDistribution=none  NoiseParameters=[]  Unit=degC  AffineConversion=on  FilteringAndDerivatives=provide  SimscapeFilterOrder=1  InputFilterTimeConstant=0.001  UdotUserProvided=0
  Transfer Fcn : TransferFcn  Denominator=[1 1]
  A : PMIOPort  Side=Right
  B : PMIOPort  Port=2  Side=Left
  wires:
  Transfer Fcn/1 -> Simulink-PS Converter1/1
  [T_stack] -> Transfer Fcn/1
  Proportional Control/1(Mw) -> Simulink-PS Converter/1
  Relative Humidity/1 -> Proportional Control/1(RH_set)
  PS-Simulink Converter/1 -> Proportional Control/2(RH_meas)
  connections:
  Controlled Moisture Source (MA)/RConn2 -- Simulink-PS Converter1/RConn1
  Measurement Selector (MA)/LConn1 -- Pipe (MA)/RConn3
  Simulink-PS Converter/RConn1 -- Controlled Moisture Source (MA)/RConn1
  Perfect Insulator/LConn1 -- Pipe (MA)/LConn2
  Measurement Selector (MA)/RConn3 -- PS-Simulink Converter/LConn1
  Controlled Moisture Source (MA)/LConn1 -- Pipe (MA)/LConn3
  Pipe (MA)/RConn1 -- B/RConn1
  Pipe (MA)/LConn1 -- A/RConn1

== system thermal_closed_loop_model/Basic Peripherals/Variant Subsystem/Controlled_Temperature_HeatExchanger/°C to Kelvin ==
  Temp. (°C) : Inport
  Constant : Constant  Value=273.15
  Sum : Sum  Inputs=|++
  Temp. (K) : Outport
  wires:
  Constant/1 -> Sum/2
  Sum/1 -> Temp. (K)/1
  Temp. (°C)/1 -> Sum/1

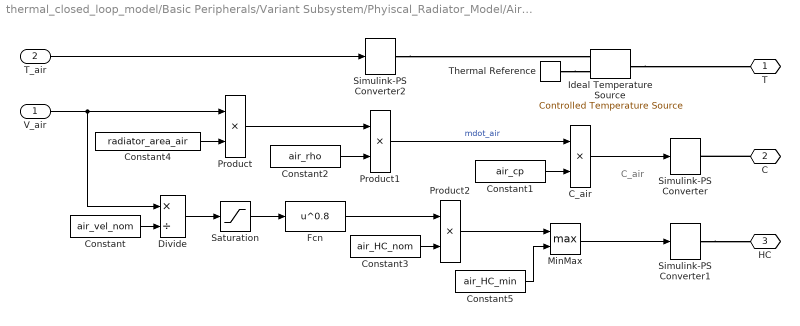
== system thermal_closed_loop_model/Basic Peripherals/Variant Subsystem/Phyiscal_Radiator_Model/Aircraft Duct ==
  note: C_air
  V_air : Inport
  T_air : Inport  Port=2
  C_air : Product
  Constant : Constant  Value=air_vel_nom
  Constant1 : Constant  Value=air_cp
  Constant2 : Constant  Value=air_rho
  Constant3 : Constant  Value=air_HC_nom
  Constant4 : Constant  Value=radiator_area_air
  Constant5 : Constant  Value=air_HC_min
  Divide : Product  Inputs=*/
  Fcn : Fcn  Expr=u^0.8
  Ideal Temperature Source : fl_lib/Thermal/Thermal Sources/Controlled Temperature Source
  MinMax : MinMax  Function=max  Inputs=2
  Product : Product
  Product1 : Product
  Product2 : Product
  Saturation : Saturate  UpperLimit=inf  LowerLimit=0
  Simulink-PS Converter : nesl_utility/Simulink-PS Converter  PhysicalDomain=network_engine_domain  SubClassName=ps_input  LeftPortType=input  RightPortType=output  PseudoPeriodic=off  Frequencies=[]  NoiseDistribution=none  NoiseParameters=[]  Unit=W/K  AffineConversion=off  FilteringAndDerivatives=zero  SimscapeFilterOrder=1  InputFilterTimeConstant=1  UdotUserProvided=1
  Simulink-PS Converter1 : nesl_utility/Simulink-PS Converter  PhysicalDomain=network_engine_domain  SubClassName=ps_input  LeftPortType=input  RightPortType=output  PseudoPeriodic=off  Frequencies=[]  NoiseDistribution=none  NoiseParameters=[]  Unit=W/(m^2*K)  AffineConversion=off  FilteringAndDerivatives=zero  SimscapeFilterOrder=1  InputFilterTimeConstant=1  UdotUserProvided=1
  Simulink-PS Converter2 : nesl_utility/Simulink-PS Converter  PhysicalDomain=network_engine_domain  SubClassName=ps_input  LeftPortType=input  RightPortType=output  PseudoPeriodic=off  Frequencies=[]  NoiseDistribution=none  NoiseParameters=[]  Unit=K  AffineConversion=on  FilteringAndDerivatives=zero  SimscapeFilterOrder=1  InputFilterTimeConstant=1  UdotUserProvided=1
  Thermal Reference : fl_lib/Thermal/Thermal Elements/Thermal Reference
  T : PMIOPort  Side=Right
  C : PMIOPort  Port=2  Side=Right
  HC : PMIOPort  Port=3  Side=Right
  wires:
  V_air/1 -> Product/1, Divide/1
  Constant/1 -> Divide/2
  Constant3/1 -> Product2/2
  Divide/1 -> Saturation/1
  Fcn/1 -> Product2/1
  Product2/1 -> MinMax/1
  Constant5/1 -> MinMax/2
  MinMax/1 -> Simulink-PS Converter1/1
  T_air/1 -> Simulink-PS Converter2/1
  Constant1/1 -> C_air/2
  C_air/1 -> Simulink-PS Converter/1
  Product/1 -> Product1/1
  Constant2/1 -> Product1/2
  Constant4/1 -> Product/2
  Product1/1 -> C_air/1  "mdot_air"
  Saturation/1 -> Fcn/1
  connections:
  C/RConn1 -- Simulink-PS Converter/RConn1
  Simulink-PS Converter1/RConn1 -- HC/RConn1
  Thermal Reference/LConn1 -- Ideal Temperature Source/RConn2
  Simulink-PS Converter2/RConn1 -- Ideal Temperature Source/RConn1
  Ideal Temperature Source/LConn1 -- T/RConn1

== system thermal_closed_loop_model/Fast Controller/CHU-Dry side control/Cathode Humidifier/Proportional Control ==
  RH_set : Inport
  RH_meas : Inport  Port=2
  Gain : Gain  Gain=0.1
  Saturation : Saturate  UpperLimit=inf  LowerLimit=0  ZeroCross=off
  Sum : Sum  Inputs=|+-
  Transfer Fcn : TransferFcn  Denominator=[1 1]
  Mw : Outport
  wires:
  Saturation/1 -> Transfer Fcn/1
  Gain/1 -> Saturation/1
  Transfer Fcn/1 -> Mw/1
  RH_meas/1 -> Sum/2
  Sum/1 -> Gain/1
  RH_set/1 -> Sum/1

== matlab function thermal_closed_loop_model/Plant_Sensors1/EAT_Theo_Power/MATLAB Function ==
  data: u input; y output; data input
function y = fcn(u, data)

y = (u^data)-1;

== matlab function thermal_closed_loop_model/Plant_Sensors1/EAC_Theo_Power/MATLAB Function ==
  data: u input; y output; data input
function y = fcn(u, data)

y = (u^data)-1;
